simulink model "FSK"  (R2017a)
settings: Solver=VariableStepAuto  StartTime=0.0  StopTime=10.0  RelTol=1e-3
libraries: dsparch4 x4, dspsrcs4 x2, simulink x1, commrandsrc3 x1, commsink2 x1
settings Model: Creator=81228  LastModifiedBy=81228

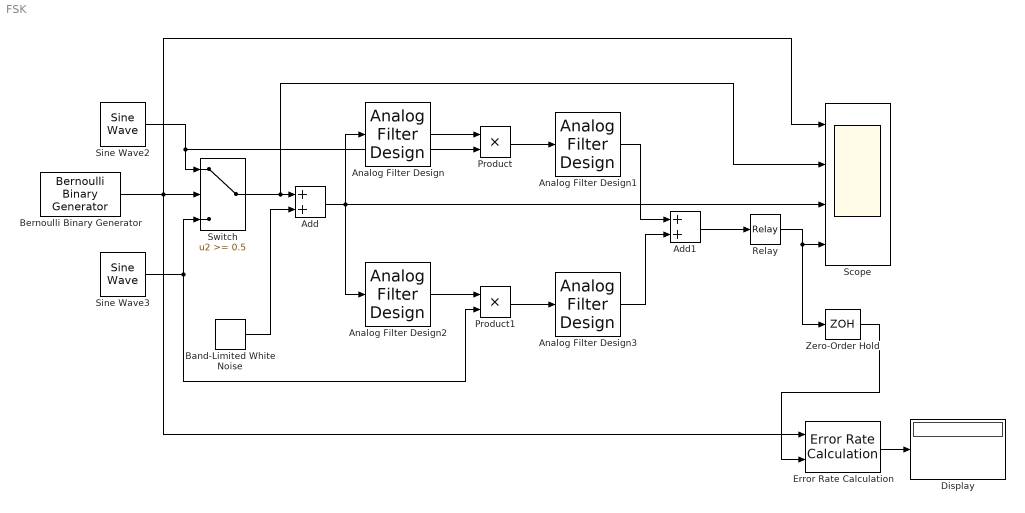
== system FSK ==
  Add : Sum
  Add1 : Sum
  Analog Filter Design : dsparch4/Analog Filter Design  method=Butterworth  filttype=Bandpass  N=8  Wlo=2*pi  Whi=10*pi  Rp=2  Rs=40
  Analog Filter Design1 : dsparch4/Analog Filter Design  method=Butterworth  filttype=Lowpass  N=8  Wlo=4*pi  Whi=26*pi  Rp=2  Rs=40
  Analog Filter Design2 : dsparch4/Analog Filter Design  method=Butterworth  filttype=Bandpass  N=8  Wlo=18*pi  Whi=26*pi  Rp=2  Rs=40
  Analog Filter Design3 : dsparch4/Analog Filter Design  method=Butterworth  filttype=Lowpass  N=8  Wlo=20*pi  Whi=80  Rp=2  Rs=40
  Band-Limited White Noise : simulink/Sources/Band-Limited White Noise  Cov=[0.001]  Ts=0.1  seed=[23341]
  Bernoulli Binary Generator : commrandsrc3/Bernoulli Binary Generator  ProbabilityOfZero=0.5  SeedSource=Parameter  Seed=61  SampleTime=1  SamplesPerFrame=1  OutputDataType=double  SimulateUsing=Interpreted execution
  Display : Display
  Error Rate Calculation : commsink2/Error Rate Calculation  N=0  st_delay=0  cp_mode=Entire frame  subframe=[]  PMode=Port  WsName=ErrorVec  RsMode2=off  stop=off  numErr=100  maxBits=1e6
  Product : Product
  Product1 : Product
  Relay : Relay
  Scope : Scope  NumInputPorts=4
  Sine Wave2 : dspsrcs4/Sine Wave  Amplitude=1  Frequency=2  Phase=0  SampleMode=Discrete  OutComplex=Real  CompMethod=Trigonometric fcn  TableSize=Speed  SampleTime=0.002  SamplesPerFrame=1  ResetState=Restart at time zero  OutputFrames=off  dataType=double  wordLen=16  udDataType=sfix(16)  fracBitsMode=Best precision  numFracBits=15  OutDataTypeStr=double  LastOutDataTypeStr=double
  Sine Wave3 : dspsrcs4/Sine Wave  Amplitude=1  Frequency=10  Phase=0  SampleMode=Discrete  OutComplex=Real  CompMethod=Trigonometric fcn  TableSize=Speed  SampleTime=0.002  SamplesPerFrame=1  ResetState=Restart at time zero  OutputFrames=off  dataType=double  wordLen=16  udDataType=sfix(16)  fracBitsMode=Best precision  numFracBits=15  OutDataTypeStr=double  LastOutDataTypeStr=double
  Switch : Switch  Threshold=0.5
  Zero-Order Hold : ZeroOrderHold
  wires:
  Switch/1 -> Scope/2, Add/1
  Sine Wave3/1 -> Product1/2, Switch/3
  Add/1 -> Scope/3, Analog Filter Design/1, Analog Filter Design2/1
  Analog Filter Design/1 -> Product/1
  Product/1 -> Analog Filter Design1/1
  Analog Filter Design2/1 -> Product1/1
  Product1/1 -> Analog Filter Design3/1
  Analog Filter Design1/1 -> Add1/1
  Analog Filter Design3/1 -> Add1/2
  Add1/1 -> Relay/1
  Relay/1 -> Zero-Order Hold/1, Scope/4
  Sine Wave2/1 -> Product/2, Switch/1
  Bernoulli Binary Generator/1 -> Scope/1, Error Rate Calculation/1, Switch/2
  Error Rate Calculation/1 -> Display/1
  Zero-Order Hold/1 -> Error Rate Calculation/2
  Band-Limited White Noise/1 -> Add/2
